simulink library "ex6lib"  (R2025b)
settings: Solver=VariableStepAuto  StartTime=0.0  StopTime=10.0  RelTol=1e-3
settings Model: Creator=fred  LastModifiedBy=fred

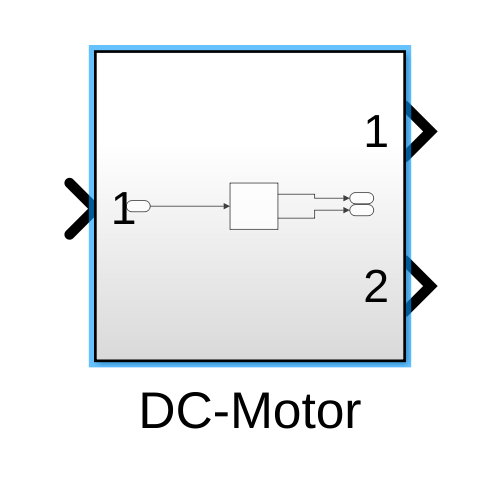
[thumbnail: Simulink's stored preview of the top-level diagram]
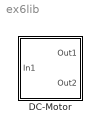
== system ex6lib ==
  DC-Motor : Subsystem

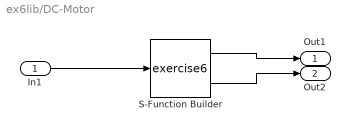
== system ex6lib/DC-Motor ==
  In1 : Inport
  S-Function Builder : S-Function  FunctionName=exercise6  Parameters=1,1,1,1,1  SFunctionModules=exercise6_wrapper.cpp  SFunctionDeploymentMode=off  EnableBusSupport=off  mask(S-Function Builder){}
      mask help: Simulink:masks:SFunctionBuilder_MD
      mask init:
      | val = [[.9  0.75 0.75 1 1 .9 .9 1]',[1 1 0.75 0.75 .9 .9 1 .9]'];try , sys = get_param(gcb,'SfunBuilderFcnName');if isempty(sys), sys = get_param(gcb,'FunctionName'); end,catch, sys = get_param(gcb,'FunctionName'); end
      settings: CopyFcn=set_param(gcbh,'LinkStatus','none')  OpenFcn=sfunctionwizard(gcbh)
      mask Display:
      | % Draw simple blue rectangle for block icon
      | rectangle('Position',[0.1 0.1 0.8 0.8], 'FaceColor',[0.5 0.8 1], 'EdgeColor','b', 'LineWidth',2);
      | 
      | % Hide axes and fix aspect ratio
      | axis off
      | xlim([0 1]); ylim([0 1]);
      | axis equal
  Out1 : Outport
  Out2 : Outport  Port=2
  wires:
  S-Function Builder/2 -> Out2/1
  In1/1 -> S-Function Builder/1
  S-Function Builder/1 -> Out1/1
